simulink model "dvlAiding"  (R2014a)
settings: Solver=ode3  StartTime=0.0  StopTime=t_stop  FixedStep=0.1  RelTol=1e-3
values from neighbouring files (symbols this model uses):
  E = E(:,1:2)    [runKalmanFilter.m]    (also in runMultiSims.m)
  G = inv(E'*E)*E'    [runKalmanFilter.m]    (also in runMultiSims.m)
  T_dvl = 600    [runKalmanFilter.m]    (also in runMultiSims.m)
  use_dvl_bias = 1    [runKalmanFilter.m]    (also in runMultiSims.m)
undefined symbols (not defined in the file or in its folder): kalman_LS, kalman_r
settings Model: Creator=mariutho  LastModifiedBy=mariutho

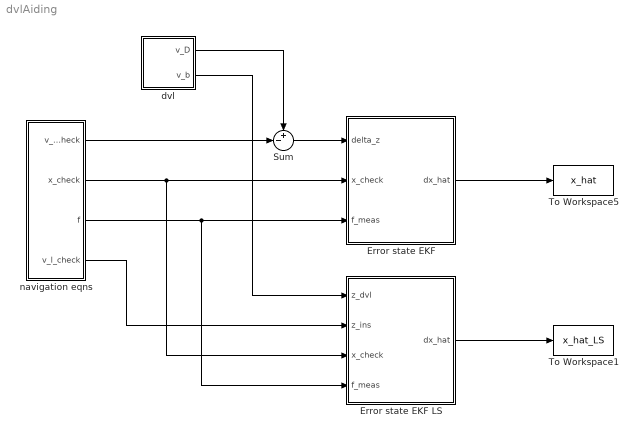
== system dvlAiding ==
  Error state EKF : Subsystem
  Error state EKF LS : Subsystem
  Sum : Sum  Inputs=+-|
  To Workspace1 : ToWorkspace  VariableName=x_hat_LS  SaveFormat=Structure  SampleTime=-1
  To Workspace5 : ToWorkspace  VariableName=x_hat  SaveFormat=Structure  SampleTime=-1
  dvl : Subsystem
  navigation eqns : Subsystem
  wires:
  navigation eqns/1(v_D_check) -> Sum/2
  navigation eqns/2(x_check) -> Error state EKF LS/3(x_check), Error state EKF/2(x_check)
  Error state EKF/1(dx_hat) -> To Workspace5/1
  Sum/1 -> Error state EKF/1(delta_z)
  dvl/1(v_D) -> Sum/1
  navigation eqns/3(f) -> Error state EKF LS/4(f_meas), Error state EKF/3(f_meas)
  navigation eqns/4(v_l_check) -> Error state EKF LS/2(z_ins)
  dvl/2(v_b) -> Error state EKF LS/1(z_dvl)
  Error state EKF LS/1(dx_hat) -> To Workspace1/1

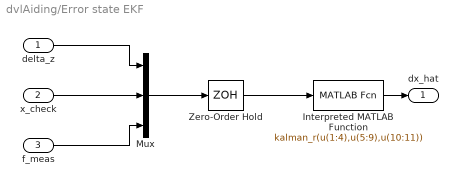
== system dvlAiding/Error state EKF ==
  delta_z : Inport
  x_check : Inport  Port=2
  f_meas : Inport  Port=3
  Interpreted MATLAB Function : MATLABFcn  MATLABFcn=kalman_r(u(1:4),u(5:9),u(10:11))
  Mux : Mux  Inputs=3
  Zero-Order Hold : ZeroOrderHold  SampleTime=0.1
  dx_hat : Outport
  wires:
  Mux/1 -> Zero-Order Hold/1
  Interpreted MATLAB Function/1 -> dx_hat/1
  f_meas/1 -> Mux/3
  delta_z/1 -> Mux/1
  x_check/1 -> Mux/2
  Zero-Order Hold/1 -> Interpreted MATLAB Function/1

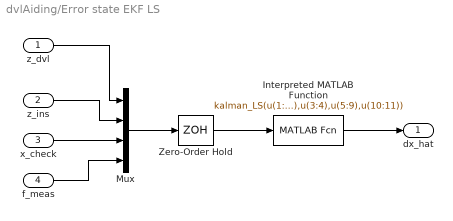
== system dvlAiding/Error state EKF LS ==
  z_dvl : Inport
  z_ins : Inport  Port=2
  x_check : Inport  Port=3
  f_meas : Inport  Port=4
  Interpreted MATLAB Function : MATLABFcn  MATLABFcn=kalman_LS(u(1:2),u(3:4),u(5:9),u(10:11))
  Mux : Mux
  Zero-Order Hold : ZeroOrderHold  SampleTime=0.1
  dx_hat : Outport
  wires:
  Mux/1 -> Zero-Order Hold/1
  Interpreted MATLAB Function/1 -> dx_hat/1
  z_dvl/1 -> Mux/1
  x_check/1 -> Mux/3
  f_meas/1 -> Mux/4
  z_ins/1 -> Mux/2
  Zero-Order Hold/1 -> Interpreted MATLAB Function/1

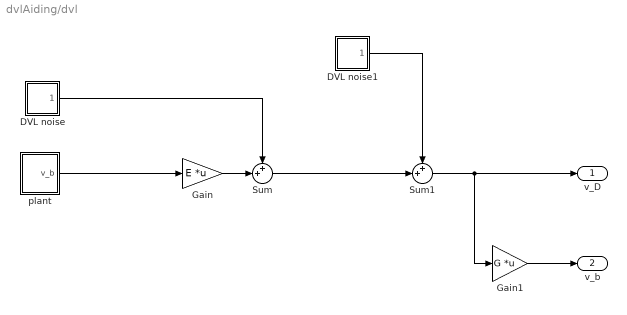
== system dvlAiding/dvl ==
  DVL noise : Subsystem
  DVL noise1 : Subsystem
  Gain : Gain  Gain=E  Multiplication=Matrix(K*u)
  Gain1 : Gain  Gain=G  Multiplication=Matrix(K*u)
  Sum : Sum  Inputs=++|
  Sum1 : Sum  Inputs=++|
  plant : Subsystem
  v_D : Outport
  v_b : Outport  Port=2
  wires:
  plant/1(v_b) -> Gain/1
  Gain/1 -> Sum/2
  DVL noise/1(delta) -> Sum/1
  Sum/1 -> Sum1/2
  Sum1/1 -> Gain1/1, v_D/1
  DVL noise1/1(delta) -> Sum1/1
  Gain1/1 -> v_b/1

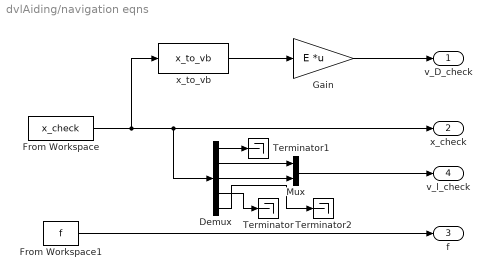
== system dvlAiding/navigation eqns ==
  Demux : Demux  Outputs=5
  From Workspace : FromWorkspace  VariableName=x_check
  From Workspace1 : FromWorkspace  VariableName=f  SampleTime=0
  Gain : Gain  Gain=E  Multiplication=Matrix(K*u)
  Mux : Mux  Inputs=2
  Terminator : Terminator
  Terminator1 : Terminator
  Terminator2 : Terminator
  x_to_vb : MATLABFcn  MATLABFcn=x_to_vb
  v_D_check : Outport
  x_check : Outport  Port=2
  f : Outport  Port=3
  v_l_check : Outport  Port=4
  wires:
  From Workspace/1 -> Demux/1, x_check/1, x_to_vb/1
  x_to_vb/1 -> Gain/1
  Gain/1 -> v_D_check/1
  From Workspace1/1 -> f/1
  Demux/2 -> Mux/1
  Demux/3 -> Mux/2
  Mux/1 -> v_l_check/1
  Demux/4 -> Terminator/1
  Demux/1 -> Terminator1/1
  Demux/5 -> Terminator2/1

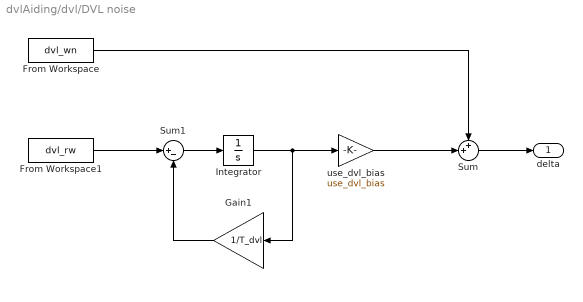
== system dvlAiding/dvl/DVL noise ==
  From Workspace : FromWorkspace  VariableName=dvl_wn  SampleTime=0
  From Workspace1 : FromWorkspace  VariableName=dvl_rw  SampleTime=0
  Gain1 : Gain  Gain=1/T_dvl
  Integrator : Integrator
  Sum : Sum  Inputs=++|
  Sum1 : Sum  Inputs=|+-
  use_dvl_bias : Gain  Gain=use_dvl_bias
  delta : Outport
  wires:
  From Workspace1/1 -> Sum1/1
  Sum1/1 -> Integrator/1
  Sum/1 -> delta/1
  use_dvl_bias/1 -> Sum/2
  Integrator/1 -> Gain1/1, use_dvl_bias/1
  Gain1/1 -> Sum1/2
  From Workspace/1 -> Sum/1

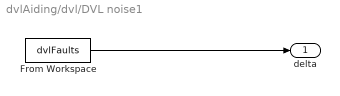
== system dvlAiding/dvl/DVL noise1 ==
  From Workspace : FromWorkspace  VariableName=dvlFaults  SampleTime=0
  delta : Outport
  wires:
  From Workspace/1 -> delta/1

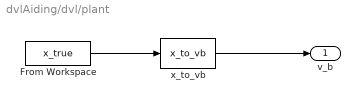
== system dvlAiding/dvl/plant ==
  From Workspace : FromWorkspace  VariableName=x_true
  x_to_vb : MATLABFcn  MATLABFcn=x_to_vb
  v_b : Outport
  wires:
  From Workspace/1 -> x_to_vb/1
  x_to_vb/1 -> v_b/1
